simulink model "Simulink_lineaire_decouple_2015a_version_ddef"  (R2015a)
settings: Solver=ode45  StartTime=0.0  StopTime=10  RelTol=1e-3
values from neighbouring files (symbols this model uses):
  A_phi = [A13_13([1 4 11],1),A13_13([1 4 11],4),A13_13([1 4 11],11)]    [SM_4.m]
  A_theta = [A13_13([2 5 12],2),A13_13([2 5 12],5),A13_13([2 5 12],12)]    [SM_4.m]
  A_z = [A13_13([3 6 13],3),A13_13([3 6 13],6),A13_13([3 6 13],13)]    [SM_4.m]
  AxS = [A13_13([7 9],7),A13_13([7 9],9)]    [SM_4.m]
  AyS = [A13_13([8 10],8),A13_13([8 10],10)]    [SM_4.m]
  B_phi = [B13_3([1 4 11],1)]    [SM_4.m]
  B_theta = [B13_3([2 5 12],2)]    [SM_4.m]
  B_z = [B13_3([3 6 13],3)]    [SM_4.m]
  BxS = [0; acc]    [SM_4.m]
  ByS = [-acc; 0]    [SM_4.m]
  C3_3_iden = eye(3)    [SM_4.m]
  C_phi = [Yd, 0, 0 ... (first row only)    [SM_4.m]
  C_theta = [-Xd, 0,0 ... (first row only)    [SM_4.m]
  C_z = [1,0,0 ... (first row only)    [SM_4.m]
  CxS = eye(2)    [SM_4.m]
  CyS = eye(2)    [SM_4.m]
  D_phi = [0;0;0]    [SM_4.m]
  D_theta = [0;0;0]    [SM_4.m]
  D_z = [0;0;0]    [SM_4.m]
  DxS = [0;0]    [SM_4.m]
  DyS = [0;0]    [SM_4.m]
  U_inv = 1/(YA*(-XB+XC)+YB*(XA-XC)+YC*(-XA+XB))*[-XB+XC, YC-YB, -YB*XC+YC*XB ... (first row only)    [SM_4.m]
  XA = r_ABC    (= 0.0952)    [SM-4.m]
  XB = -r_ABC*sind(30)    [SM-4.m]
  XC = 0    [SM-4.m]
  YA = 0    [SM-4.m]
  YB = r_ABC*cosd(30)    [SM-4.m]
  YC = -r_ABC*cosd(30)    [SM-4.m]
undefined symbols (not defined in the file or in its folder): ia_e, ib_e, ic_e, phi_e, TABC_trans, TDEF_inv, TDEF_trans, theta_e, va_e, vb_e, vc_e, vx_s_e, vy_s_e, vz_e, w_phi_e, w_theta_e, x_s_e, y_s_e, z_e
settings Model: Creator=Julien  LastModifiedBy=Julien

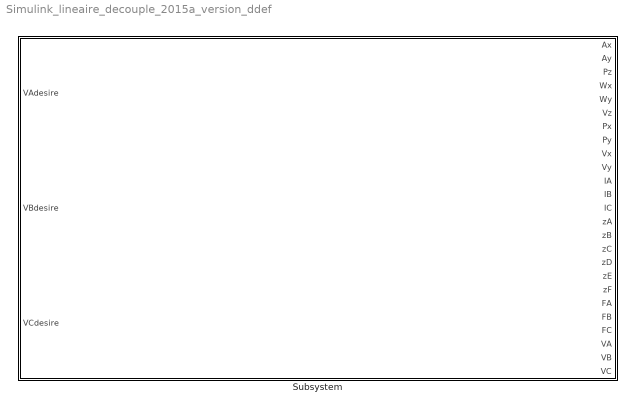
== system Simulink_lineaire_decouple_2015a_version_ddef ==
  Subsystem : Subsystem

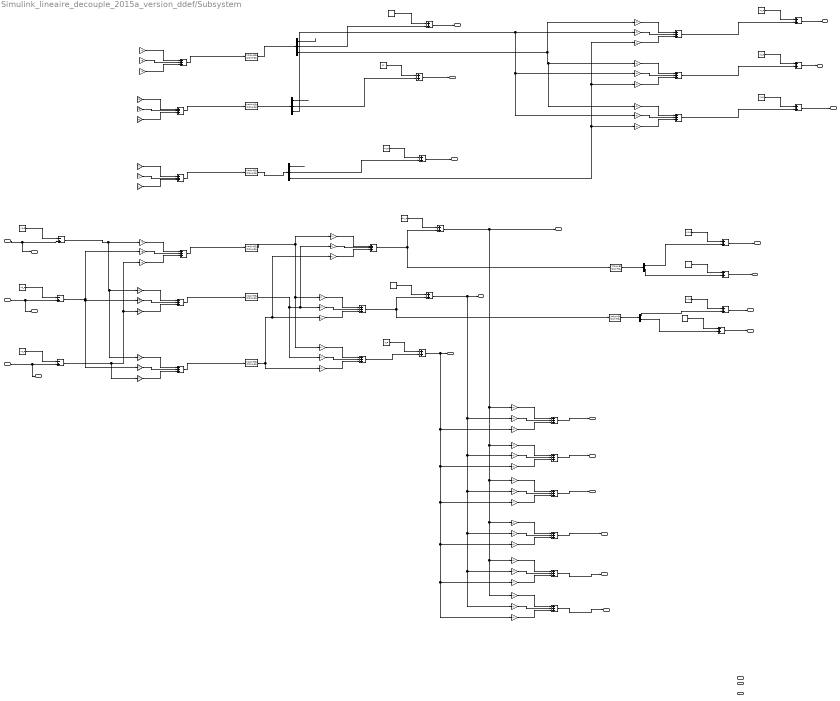
== system Simulink_lineaire_decouple_2015a_version_ddef/Subsystem ==
  note: za
  note: axe_x
  note: axe_y
  note: delta_phi
  note: delta_w_z
  note: delta_z_2
  note: delta_i_theta
  note: delta_theta_2
  note: delta_phi_2
  note: delta_phi
  note: delta_dd
  note: delat_df
  note: delta_vb
  note: delta_vphi
  note: delta_vtheta
  note: delta_vz
  note: delta_z
  note: delta_theta
  note: bus_phi
  note: delat_df
  note: delta_vphi
  note: delta_vtheta
  note: delta_vz
  note: zb
  note: zc
  note: zd
  note: ze
  note: zf
  VAdesire : Inport
  VBdesire : Inport  Port=2
  VCdesire : Inport  Port=3
  Add : Sum  Inputs=-+
  Add1 : Sum  Inputs=-+
  Add{3..12,15..16,28..33} (18 alike) : Sum  Inputs=+++
  Add{13..14,17..27} (13 alike) : Sum
  Add2 : Sum  Inputs=-+
  Constant : Constant  Value=va_e
  Constant1 : Constant  Value=vb_e
  Constant10 : Constant  Value=z_e
  Constant11 : Constant  Value=vz_e
  Constant12 : Constant  Value=vy_s_e
  Constant13 : Constant  Value=y_s_e
  Constant14 : Constant  Value=x_s_e
  Constant15 : Constant  Value=vx_s_e
  Constant2 : Constant  Value=vc_e
  Constant3 : Constant  Value=ia_e
  Constant4 : Constant  Value=w_theta_e
  Constant5 : Constant  Value=w_phi_e
  Constant6 : Constant  Value=ib_e
  Constant7 : Constant  Value=ic_e
  Constant8 : Constant  Value=phi_e
  Constant9 : Constant  Value=theta_e
  Demux : Demux  Outputs=3
  Demux1 : Demux  Outputs=3
  Demux2 : Demux  Outputs=3
  Demux3 : Demux  Outputs=2
  Demux4 : Demux  Outputs=2
  Gain : Gain  Gain=YA
  Gain1 : Gain  Gain=YB
  Gain10 : Gain  Gain=TDEF_inv(1,2)
  Gain11 : Gain  Gain=TDEF_inv(1,3)
  Gain12 : Gain  Gain=TDEF_inv(3,2)
  Gain13 : Gain  Gain=TDEF_inv(3,3)
  Gain14 : Gain  Gain=TDEF_inv(3,1)
  Gain15 : Gain  Gain=TDEF_inv(2,2)
  Gain16 : Gain  Gain=TDEF_inv(2,3)
  Gain17 : Gain  Gain=TDEF_inv(1,1)
  Gain18 : Gain  Gain=YA
  Gain19 : Gain  Gain=YB
  Gain2 : Gain  Gain=YC
  Gain20 : Gain  Gain=YC
  Gain21 : Gain  Gain=-XA
  Gain22 : Gain  Gain=-XB
  Gain23 : Gain  Gain=-XC
  Gain{6..8,24..26} (6 alike) : Gain
  Gain27 : Gain  Gain=U_inv(1,1)
  Gain28 : Gain  Gain=U_inv(1,2)
  Gain29 : Gain  Gain=U_inv(1,3)
  Gain3 : Gain  Gain=-XA
  Gain30 : Gain  Gain=U_inv(2,1)
  Gain31 : Gain  Gain=U_inv(2,2)
  Gain32 : Gain  Gain=U_inv(2,3)
  Gain33 : Gain  Gain=U_inv(3,1)
  Gain34 : Gain  Gain=U_inv(3,2)
  Gain35 : Gain  Gain=U_inv(3,3)
  Gain36 : Gain  Gain=TABC_trans(1,1)
  Gain37 : Gain  Gain=TABC_trans(1,2)
  Gain38 : Gain  Gain=TABC_trans(1,3)
  Gain39 : Gain  Gain=TABC_trans(2,1)
  Gain4 : Gain  Gain=-XB
  Gain40 : Gain  Gain=TABC_trans(2,2)
  Gain41 : Gain  Gain=TABC_trans(2,3)
  Gain42 : Gain  Gain=TABC_trans(3,1)
  Gain43 : Gain  Gain=TABC_trans(3,2)
  Gain44 : Gain  Gain=TABC_trans(3,3)
  Gain45 : Gain  Gain=TDEF_trans(1,1)
  Gain46 : Gain  Gain=TDEF_trans(1,2)
  Gain47 : Gain  Gain=TDEF_trans(1,3)
  Gain48 : Gain  Gain=TDEF_trans(2,1)
  Gain49 : Gain  Gain=TDEF_trans(2,2)
  Gain5 : Gain  Gain=-XC
  Gain50 : Gain  Gain=TDEF_trans(2,3)
  Gain51 : Gain  Gain=TDEF_trans(3,1)
  Gain52 : Gain  Gain=TDEF_trans(3,2)
  Gain53 : Gain  Gain=TDEF_trans(3,3)
  Gain9 : Gain  Gain=TDEF_inv(1,1)
  State-Space_phi : StateSpace  A=A_phi  B=B_phi  C=C_phi  D=D_phi  X0=0
  State-Space_phi1 : StateSpace  A=A_phi  B=B_phi  C=C3_3_iden  D=D_phi  X0=0
  State-Space_theta : StateSpace  A=A_theta  B=B_theta  C=C_theta  D=D_theta  X0=0
  State-Space_theta1 : StateSpace  A=A_theta  B=B_theta  C=C3_3_iden  D=D_theta  X0=0
  State-Space_xs : StateSpace  A=AxS  B=BxS  C=CxS  D=DxS  X0=0
  State-Space_ys : StateSpace  A=AyS  B=ByS  C=CyS  D=DyS  X0=0
  "State-Space_z " : StateSpace  A=A_z  B=B_z  C=C_z  D=D_z  X0=0
  State-Space_z 1 : StateSpace  A=A_z  B=B_z  C=C3_3_iden  D=D_z  X0=0
  Ax : Outport
  Ay : Outport  Port=2
  Pz : Outport  Port=3
  Wx : Outport  Port=4
  Wy : Outport  Port=5
  Vz : Outport  Port=6
  Px : Outport  Port=7
  Py : Outport  Port=8
  Vx : Outport  Port=9
  Vy : Outport  Port=10
  IA : Outport  Port=11
  IB : Outport  Port=12
  IC : Outport  Port=13
  zA : Outport  Port=14
  zB : Outport  Port=15
  zC : Outport  Port=16
  zD : Outport  Port=17
  zE : Outport  Port=18
  zF : Outport  Port=19
  FA : Outport  Port=20
  FB : Outport  Port=21
  FC : Outport  Port=22
  VA : Outport  Port=23
  VB : Outport  Port=24
  VC : Outport  Port=25
  wires:
  Constant/1 -> Add/1
  VAdesire/1 -> VA/1, Add/2
  Constant2/1 -> Add2/1
  VCdesire/1 -> VC/1, Add2/2
  Constant1/1 -> Add1/1
  VBdesire/1 -> VB/1, Add1/2
  Gain/1 -> Add3/1
  Gain1/1 -> Add3/2
  Gain2/1 -> Add3/3
  Add3/1 -> State-Space_phi/1
  Add2/1 -> Gain8/1, Gain5/1, Gain2/1  "delta_vc"
  Gain3/1 -> Add4/1
  Gain4/1 -> Add4/2
  Gain5/1 -> Add4/3
  Add4/1 -> State-Space_theta/1
  Add/1 -> Gain6/1, Gain3/1, Gain/1  "delta_va"
  Add1/1 -> Gain7/1, Gain4/1, Gain1/1  "delta_vb"
  Gain6/1 -> Add5/1
  Gain7/1 -> Add5/2
  Gain8/1 -> Add5/3
  Add5/1 -> "State-Space_z "/1
  State-Space_phi/1 -> Gain9/1, Gain17/1, Gain14/1  "delta_dd"
  State-Space_theta/1 -> Gain10/1, Gain15/1, Gain12/1  "delta_de"
  "State-Space_z "/1 -> Gain13/1, Gain11/1, Gain16/1  "delta_df"
  Gain9/1 -> Add6/1
  Gain10/1 -> Add6/2
  Gain11/1 -> Add6/3
  Gain14/1 -> Add7/1
  Gain12/1 -> Add7/2
  Gain13/1 -> Add7/3
  Add7/1 -> Add23/2
  Gain17/1 -> Add8/1
  Gain15/1 -> Add8/2
  Gain16/1 -> Add8/3
  ? -> Gain18/1  "delta_va"
  ? -> Gain19/1  "delta_vb"
  ? -> Gain20/1  "delta_vc"
  Gain18/1 -> Add9/1
  Gain19/1 -> Add9/2
  Gain20/1 -> Add9/3
  Add9/1 -> State-Space_phi1/1
  ? -> Gain21/1  "delta_va"
  ? -> Gain22/1  "delta_vb"
  ? -> Gain23/1  "delta_vc"
  Gain21/1 -> Add10/1
  Gain22/1 -> Add10/2
  Gain23/1 -> Add10/3
  Add10/1 -> State-Space_theta1/1
  ? -> Gain24/1  "delta_va"
  ? -> Gain25/1  "delta_vb"
  ? -> Gain26/1  "delta_vc"
  Gain24/1 -> Add11/1
  Gain25/1 -> Add11/2
  Gain26/1 -> Add11/3
  Add11/1 -> State-Space_z 1/1
  State-Space_phi1/1 -> Demux/1
  State-Space_theta1/1 -> Demux1/1  "delta_de"
  State-Space_z 1/1 -> Demux2/1
  Demux/2 -> Add14/2  "delta_w_phi"
  Demux1/1 -> ?
  Demux1/2 -> Add13/2  "delta_w_theta"
  Demux2/1 -> ?
  Demux2/2 -> Add20/2
  Constant4/1 -> Add13/1
  Constant5/1 -> Add14/1
  Constant11/1 -> Add20/1
  Add14/1 -> Wx/1
  Add13/1 -> Wy/1
  Add20/1 -> Vz/1
  Gain27/1 -> Add12/1
  Gain28/1 -> Add12/2
  Gain29/1 -> Add12/3
  Add12/1 -> Add17/2  "delta_ia"
  Gain30/1 -> Add15/1
  Gain31/1 -> Add15/2
  Gain32/1 -> Add15/3
  Add15/1 -> Add18/2  "delta_ib"
  Gain33/1 -> Add16/1
  Gain34/1 -> Add16/2
  Gain35/1 -> Add16/3
  Add16/1 -> Add19/2  "delta_ic"
  Demux/3 -> Gain27/1, Gain33/1, Gain30/1  "delta_i_phi"
  Demux1/3 -> Gain31/1, Gain34/1, Gain28/1  "delta_i_theta"
  Demux2/3 -> Gain35/1, Gain32/1, Gain29/1  "delta_i_z"
  Constant3/1 -> Add17/1
  Constant6/1 -> Add18/1
  Constant7/1 -> Add19/1
  Add17/1 -> IA/1
  Add18/1 -> IB/1
  Add19/1 -> IC/1
  Demux/1 -> ?
  Constant8/1 -> Add21/1
  Constant9/1 -> Add22/1
  Constant10/1 -> Add23/1
  Add6/1 -> Add21/2, State-Space_xs/1
  State-Space_xs/1 -> Demux3/1
  Add8/1 -> Add22/2, State-Space_ys/1  "delta_theta"
  State-Space_ys/1 -> Demux4/1
  Demux3/1 -> Add25/2  "delta_ys"
  Demux3/2 -> Add24/2  "dela_vys"
  Demux4/1 -> Add26/2  "delta_xs"
  Demux4/2 -> Add27/2  "delta_vxs"
  Constant12/1 -> Add24/1
  Constant13/1 -> Add25/1
  Constant14/1 -> Add26/1
  Constant15/1 -> Add27/1
  Add25/1 -> Py/1
  Add24/1 -> Vy/1
  Add26/1 -> Px/1
  Add27/1 -> Vx/1
  Gain36/1 -> Add28/1
  Gain37/1 -> Add28/2
  Gain38/1 -> Add28/3
  Add28/1 -> zA/1
  Gain39/1 -> Add29/1
  Gain40/1 -> Add29/2
  Gain41/1 -> Add29/3
  Add29/1 -> zB/1
  Gain42/1 -> Add30/1
  Gain43/1 -> Add30/2
  Gain44/1 -> Add30/3
  Add30/1 -> zC/1
  Gain45/1 -> Add31/1
  Gain46/1 -> Add31/2
  Gain47/1 -> Add31/3
  Add31/1 -> zD/1
  Gain48/1 -> Add32/1
  Gain49/1 -> Add32/2
  Gain50/1 -> Add32/3
  Add21/1 -> Gain39/1, Gain42/1, Gain45/1, Gain48/1, Gain51/1, Gain36/1, Ax/1  "phi"
  Add32/1 -> zE/1
  Gain51/1 -> Add33/1
  Gain52/1 -> Add33/2
  Gain53/1 -> Add33/3
  Add22/1 -> Gain37/1, Gain52/1, Gain49/1, Gain46/1, Gain43/1, Gain40/1, Ay/1  "theta"
  Add23/1 -> Gain38/1, Gain41/1, Gain53/1, Gain50/1, Gain47/1, Gain44/1, Pz/1  "z"
  Add33/1 -> zF/1
